simulink model "MontajeFinal"  (R2023a)
settings: Solver=ode4  StartTime=0.0  StopTime=1527  FixedStep=Ts  RelTol=1e-3  EnableMultiTasking=on
PostLoadFcn:
  | Ts=1/200000;L=1.8e-3;w=2*pi*60;C=20e-6;
  | 
  | load('NewCycleFTP75.mat')
  | 
  | Vel=Cycle(:,1);
  | Acc=Cycle(:,2);
InitFcn:
  | Ts=1/200000;L=1.8e-3;w=2*pi*60;C=20e-6;
  | 
  | load('NewCycleFTP75.mat')
  | 
  | Vel=Cycle(:,1);
  | Acc=Cycle(:,2);
values from neighbouring files (symbols this model uses):
  Cycle = [0 0 0 0 0 0 0 0 0 0 0 0 ... (4948 elements, 2474x2)]    [CycleFTP75.mat]    (also in CycleOntibon.mat = [0 0 0 0 0 0 0 0 0 0 0 0 ... (3602 elements, 1801x2)])
undefined symbols (not defined in the file or in its folder): DiscIntNeverNeededParam, sizecont
libraries: simulink x10, spsSeriesRLCBranchLib x8, spsIGBTDiodeLib x6, spsCurrentMeasurementLib x4, spsVoltageMeasurementLib x4, spsGroundLib x4, dspswit3 x2, spsDCVoltageSourceLib x1, spsAsynchronousMachineSIUnitsLib x1, spspowerguiLib x1, slpidlib x1
(part 1 of 2)
Description:
  | Model of a simple control system for use iin training.
settings Model: SimulationMode=accelerator  Creator=Paul Baracos  LastModifiedBy=Julian
settings SolverCC: AlgebraicLoopSolver=TrustRegion
settings DataIOCC: LimitDataPoints=on  SaveFormat=Array  SignalLoggingSaveFormat=ModelDataLogs  SaveOutput=off  SaveTime=off  ReturnWorkspaceOutputs=off  SignalLoggingName=sigsOut
settings OptimizationCC: BlockReduction=off  BooleanDataType=off  OptimizeBlockIOStorage=off  BufferReuse=off  ReuseModelBlockBuffer=off  GlobalBufferReuse=off  ExpressionFolding=off  LocalBlockOutputs=off  InitFltsAndDblsToZero=on  LifeSpan=inf
settings DebuggingCC: SaveWithParameterizedLinksMsg=none  UnderspecifiedInitializationDetection=Classic  MergeDetectMultiDrivingBlocksExec=none  SignalResolutionControl=TryResolveAllWithWarning  MultiTaskDSMMsg=warning  MultiTaskCondExecSysMsg=none  FcnCallInpInsideContextMsg=warning  UnconnectedInputMsg=warning  UnconnectedOutputMsg=warning  UnconnectedLineMsg=warning  SFUnexpectedBacktrackingDiag=warning  SFNoUnconditionalDefaultTransitionDiag=warning  SFExecutionAtInitializationDiag=none  ArithmeticOperatorsInVariantConditions=warning
settings HardwareCC: ProdBitPerPointer=32  ProdBitPerSizeT=32  ProdBitPerPtrDiffT=32  ProdLargestAtomicFloat=None  ProdIntDivRoundTo=Undefined  ProdEndianess=Unspecified  ProdWordSize=32  ProdHWDeviceType=32-bit Generic  TargetUnknown=on
settings ModelReferenceCC: EnableRefExpFcnMdlSchedulingChecks=on  PropagateSignalLabelsOutOfModel=off
settings SFSimCC: SimUseLocalCustomCode=off  CustomCodeUndefinedFunction=UseInterfaceOnly
settings RTWCC: RTWUseLocalCustomCode=off
settings CodeAppCC: StateflowObjectComments=on
settings GRTTargetCC: TargetFcnLib=ansi_tfl_tmw.mat  TargetLangStandard=C89/C90 (ANSI)  CombineOutputUpdateFcns=off  GRTInterface=on
settings ConfigComp: CovMetricSettings=dw  CovSaveCumulativeToWorkspaceVar=on  CovSaveSingleToWorkspaceVar=on  CovExternalEMLEnable=off
settings SimscapeCC: SimscapeNormalizeSystem=off

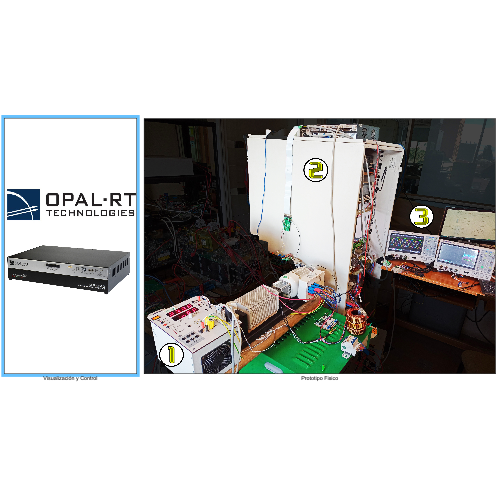
[thumbnail: Simulink's stored preview of the top-level diagram]
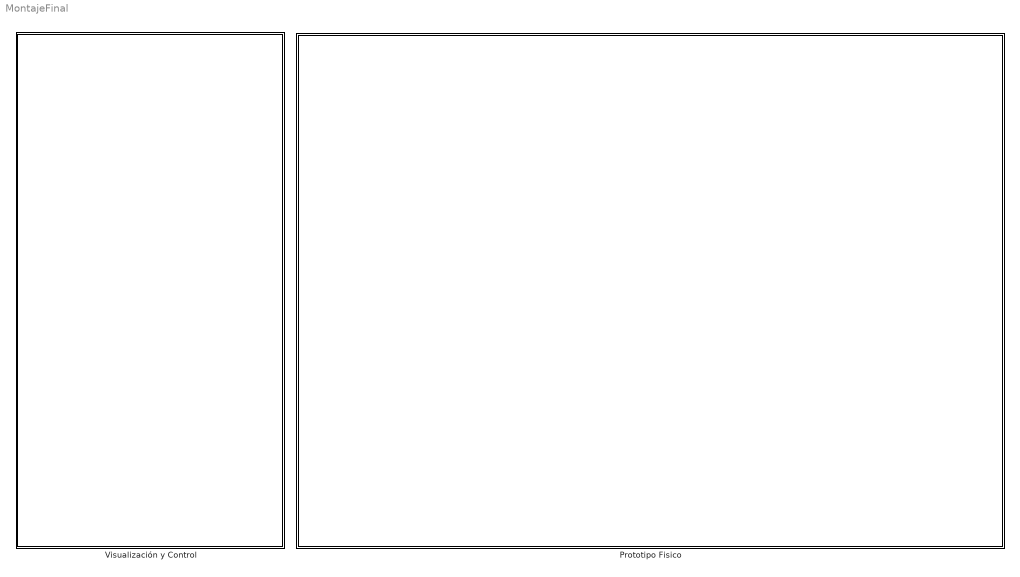
== system MontajeFinal ==
  Prototipo Fisico : Subsystem
      mask Display: image('General.jpg'); % Use "Edit Image" on toolstrip to change.
  Visualización y Control : Subsystem
      mask Display: image('Opal.jpg'); % Use "Edit Image" on toolstrip to change.

== system MontajeFinal/Prototipo Fisico ==
  Fuente Bidireccional : Subsystem
      mask Display: image('Fuente.jpg'); % Use "Edit Image" on toolstrip to change.
  Inversor - Filtro LC - Sensores : Subsystem
      mask Display: image('Sensores.jpg'); % Use "Edit Image" on toolstrip to change.
  Maquina Pendular & MIJA : Subsystem
      mask Display: image('Maquinas.jpg'); % Use "Edit Image" on toolstrip to change.
  Modulo Comunicación : Subsystem
      settings: PortSchema="{\"entries\":[{\"content\":{\"sides\":[{\"content\":{\"connectorIds\":[\"Out2\",\"In1\"]},\"type\":\"ConnectorPlacement.EquallySpacedRectSide\",\"uuid\":\"66e5c735-c63b-4ba9-ad41-caef14ec7bf0\"},{\"content\":{\"connectorIds\":[\"In2\",\"Out1\"],\"side\":\"RIGHT\"},\"type\":\"ConnectorPlacement.EquallySpacedRectSide\",\"uuid\":\"f3b04e68-f383-44b7-b279-598a5bf2e637\"},{\"content\":{\"side\":\"TOP\"},\"type\":\"ConnectorPlacement.EquallySpacedRectSide\",\"uuid\":\"c3216178-39f9-4474-948a-42e4050edd7e\"}]},\"type\":\"ConnectorPlacement.EquallySpacedConnector\",\"uuid\":\"a4194594-47fb-4665-9fd1-3f005c2be821\"}],\"packageUris\":[\"http://schema.mathworks.com/mf0/Connector/R2020b\"],\"version\":\"1.0\"}"
      mask Display: image('G:\Mi unidad\VEHICULO ELECTRICO\Articulos\Simposios\Sicel\Imagenes\Final\Comunicacion.jpg'); % Use "Edit Image" on toolstrip to change.
  powergui : spspowerguiLib/powergui  Priority=1  SimulationMode=Discrete  SampleTime=Ts  frequency=60  Iterations=50  frequencyindice=0  Pbase=100e6  ErrMax=1e-4  UnitsV=kV  UnitsW=MW  buscounter=0  FunctionMessages=off  echomessages=off  EnableUseOfTLC=off  CurrentSourceSwitches=off  DisableSnubberDevices=off  DisableRonSwitches=off  DisableVfSwitches=off  DisplayEquations=off  AutomaticDiscreteSolvers=off  SolverType=Tustin/Backward Euler (TBE)  Interpol=off  ExternalGateDelay=off  methode=off  Ts=100  x0status=blocks  SPID=on  SwTol=0  HookPort=off  NonlinearTolerance=1e-4  nMaxIteration=100  ContinueOnMaxIteration=off  RestoreLinks=warning  ResistiveCurrentMeasurement=off  Frange=[0:2:500]  Ylog=off  Xlog=on  ShowGrid=off  save=off  variable=ZData  structure=0  ZoomFFT=off  StartTime=0.0  cycles=1  DisplayStyle=1  fundamental=60  FreqAxis=off  MaxFrequency=1000  frequencyindicesteady=1  RmsSteady=1  display=off
  tag scope: Velocidad=global
  wires:
  Modulo Comunicación/1(Par_Out) -> Maquina Pendular & MIJA/1(Par)
  Modulo Comunicación/2(Vel_Out) -> [Velocidad]
  [Par] -> Modulo Comunicación/1(Par_In)
  Maquina Pendular & MIJA/1(Velocidad) -> Modulo Comunicación/2(Vel_In)
  connections:
  Fuente Bidireccional/RConn1 -- Inversor - Filtro LC - Sensores/LConn1
  Inversor - Filtro LC - Sensores/RConn2 -- Maquina Pendular & MIJA/LConn2
  Inversor - Filtro LC - Sensores/RConn3 -- Maquina Pendular & MIJA/LConn3
  Fuente Bidireccional/RConn2 -- Inversor - Filtro LC - Sensores/LConn2
  Inversor - Filtro LC - Sensores/RConn1 -- Maquina Pendular & MIJA/LConn1

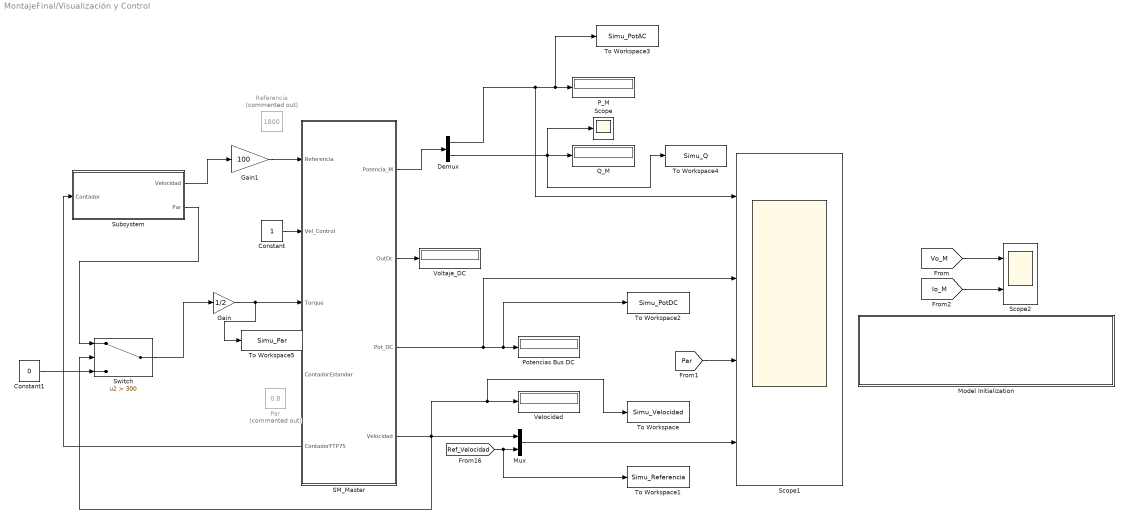
== system MontajeFinal/Visualización y Control ==
  Constant : Constant
  Constant1 : Constant  Value=0
  Demux : Demux  Outputs=2
  Gain : Gain  Gain=1/2
  Gain1 : Gain  Gain=100  SaturateOnIntegerOverflow=on  OutDataTypeStr=Inherit: Same as input  ParamDataTypeStr=Inherit: Same as input
  Model Initialization : Subsystem  AncestorBlock=artemis/Tools /Misc/Model Initialization  mask(Model Functions){InitFcnX=|, prel=off, posl=on, inif=on, strf=off}
      mask InitFcnX=|
      | Ts=1/200000;L=1.8e-3;w=2*pi*60;C=20e-6;
      |
      | load('NewCycleFTP75.mat')
      |
      | Vel=Cycle(:,1);
      | Acc=Cycle(:,2);
      mask prompts: InitFcnX "Initialisation"; prel "Preload Function"; posl "PostLoad Function"; inif "InitFcn"; strf "StartFcn"
      mask init:
      | currentBlock = gcb;
      | root = bdroot(currentBlock);
      | 
      | if ~strcmp(get_param(root,'BlockDiagramType'),'library')
      |     if prel==1
      |         set_param(root, 'PreLoadFcn', InitFcnX);
      |     else
      |         set_param(root, 'PreLoadFcn', '');
      |     end
      |     if inif==1
      |         set_param(root, 'InitFcn', InitFcnX);
      |     else
      |         set_param(root, 'InitFcn', '');
      |     end
      |     if strf==1
      |         set_param(root, 'StartFcn', InitFcnX);
      |     else
      |         set_param(root, 'StartFcn', '');
      |     end
      |     if posl==1
      |         set_param(root, 'PostLoadFcn', InitFcnX);
      |     else
      |         set_param(root, 'PostLoadFcn', '');
      |     end
      | end
      | 
      | pos = get_param(currentBlock, 'Position');
      | width = pos(3) - pos(1); height = pos(4) - pos(2);
      | txt = [ upper(root) '\n' '- InitFcn. . . . . '  get_param(root, 'InitFcn') ];
      settings: LibrarySourceBlock=artemis/Tools /Misc/Model Initialization  CopyFcn=set_param(gcb,'LinkStatus','inactive')
      mask Display: text(5, height*0.5, txt, 'horizontalAlignment', 'left', 'verticalAlignment', 'middle') ;
  Mux : Mux  Inputs=2
  P_M : Display
  Par : Constant  Commented=on  Value=0.8
  Potencias Bus DC : Display
  Q_M : Display
  Referencia : Constant  Commented=on  Value=1800
  SM_Master : Subsystem
      settings: PortSchema="{\"entries\":[{\"content\":{\"sides\":[{\"content\":{\"connectorIds\":[\"In1\",\"In2\",\"In3\",\"Out5\",\"Out6\"]},\"type\":\"ConnectorPlacement.EquallySpacedRectSide\",\"uuid\":\"2bfde8e4-db29-467b-a3e6-219bd979e2b6\"},{\"content\":{\"connectorIds\":[\"Out1\",\"Out2\",\"Out3\",\"Out4\"],\"side\":\"RIGHT\"},\"type\":\"ConnectorPlacement.EquallySpacedRectSide\",\"uuid\":\"a7f0eab7-0a0b-47e1-a185-527893d455d2\"},{\"content\":{\"side\":\"TOP\"},\"type\":\"ConnectorPlacement.EquallySpacedRectSide\",\"uuid\":\"1aba6232-4c2d-4fe6-89ed-3e8cc09b7475\"}]},\"type\":\"ConnectorPlacement.EquallySpacedConnector\",\"uuid\":\"12a0442f-195f-492e-b9e3-ea8deb1e0ede\"}],\"packageUris\":[\"http://schema.mathworks.com/mf0/Connector/R2020b\"],\"version\":\"1.0\"}"
  Scope : Scope
  Scope1 : Scope  NumInputPorts=4
  Scope2 : Scope  NumInputPorts=2
  Subsystem : Subsystem
  Switch : Switch  Criteria=u2 > Threshold  Threshold=300  SaturateOnIntegerOverflow=off  InputSameDT=off
  To Workspace : ToWorkspace  VariableName=Simu_Velocidad  SampleTime=1/2000
      settings: Save2DSignal=2-D array (concatenate along first dimension)
  To Workspace1 : ToWorkspace  VariableName=Simu_Referencia  SampleTime=1/2000
      settings: Save2DSignal=2-D array (concatenate along first dimension)
  To Workspace2 : ToWorkspace  VariableName=Simu_PotDC  SampleTime=1/2000
      settings: Save2DSignal=2-D array (concatenate along first dimension)
  To Workspace3 : ToWorkspace  VariableName=Simu_PotAC  SampleTime=1/2000
      settings: Save2DSignal=2-D array (concatenate along first dimension)
  To Workspace4 : ToWorkspace  VariableName=Simu_Q  SampleTime=1/2000
      settings: Save2DSignal=2-D array (concatenate along first dimension)
  To Workspace5 : ToWorkspace  VariableName=Simu_Par  SampleTime=1/2000
      settings: Save2DSignal=2-D array (concatenate along first dimension)
  Velocidad : Display
  Voltaje_DC : Display
  wires:
  SM_Master/1(Potencia_M) -> Demux/1
  Demux/2 -> To Workspace4/1, Scope/1, Q_M/1
  Demux/1 -> Scope1/1, To Workspace3/1, P_M/1
  SM_Master/2(OutDc) -> Voltaje_DC/1
  Constant/1 -> SM_Master/2(Vel_Control)
  SM_Master/3(Pot_DC) -> To Workspace2/1, Potencias Bus DC/1, Scope1/2
  SM_Master/4(Velocidad) -> Switch/2, To Workspace/1, Velocidad/1, Mux/1
  [Ref_Velocidad] -> To Workspace1/1, Mux/2
  [Vo_M] -> Scope2/1
  [Io_M] -> Scope2/2
  [Par] -> Scope1/3
  Mux/1 -> Scope1/4
  Gain/1 -> To Workspace5/1, SM_Master/3(Torque)
  SM_Master/6(ContadorFTP75) -> Subsystem/1(Contador)
  Gain1/1 -> SM_Master/1(Referencia)
  Subsystem/1(Velocidad) -> Gain1/1
  Switch/1 -> Gain/1
  Constant1/1 -> Switch/3
  Subsystem/2(Par) -> Switch/1

== system MontajeFinal/Prototipo Fisico/Fuente Bidireccional ==
  Current Measurement3 : spsCurrentMeasurementLib/Current Measurement  PhasorSimulation=off  OutputType=Complex  PSBequivalent=0
  DC Voltage Source : spsDCVoltageSourceLib/DC Voltage Source  Amplitude=1000  Measurements=None
  Series RLC Branch6 : spsSeriesRLCBranchLib/Series RLC Branch  LConnTagsString=__new0  RConnTagsString=__new0  BranchType=C  Resistance=0.0000000000000000000000000000000000000000000001  Inductance=L  SetiL0=off  InitialCurrent=0  Capacitance=0.1  Setx0=off  InitialVoltage=0  Measurements=None
  Series RLC Branch7 : spsSeriesRLCBranchLib/Series RLC Branch  LConnTagsString=__new0  RConnTagsString=__new0  BranchType=R  Resistance=0.1  Inductance=L  SetiL0=off  InitialCurrent=0  Capacitance=0.001  Setx0=off  InitialVoltage=0  Measurements=None
  Voltage Measurement4 : spsVoltageMeasurementLib/Voltage Measurement  PhasorSimulation=off  OutputType=Complex  PSBequivalent=0
  + : PMIOPort  Side=Right
  - : PMIOPort  Port=2  Side=Right
  tag scope: Idc=global, Vdc=global
  wires:
  Voltage Measurement4/1 -> [Vdc]
  Current Measurement3/1 -> [Idc]
  connections:
  Series RLC Branch7/LConn1 -- Series RLC Branch6/LConn1 -- Voltage Measurement4/LConn1 -- +/RConn1
  Series RLC Branch6/RConn1 -- DC Voltage Source/LConn1 -- -/RConn1 -- Voltage Measurement4/LConn2
  Series RLC Branch7/RConn1 -- Current Measurement3/RConn1
  Current Measurement3/LConn1 -- DC Voltage Source/RConn1

== system MontajeFinal/Prototipo Fisico/Inversor - Filtro LC - Sensores ==
  Filtro LC & Sensores : Subsystem
  Inversor : Subsystem
  a : PMIOPort  Side=Right
  Vdc : PMIOPort  Port=2  Side=Left
  b : PMIOPort  Port=3  Side=Right
  -Vdc : PMIOPort  Port=4  Side=Left
  c : PMIOPort  Port=5  Side=Right
  connections:
  Filtro LC & Sensores/LConn3 -- Inversor/RConn3
  Filtro LC & Sensores/LConn1 -- Inversor/RConn1
  Filtro LC & Sensores/RConn2 -- b/RConn1
  Filtro LC & Sensores/LConn2 -- Inversor/RConn2
  Filtro LC & Sensores/RConn1 -- a/RConn1
  Filtro LC & Sensores/RConn3 -- c/RConn1
  -Vdc/RConn1 -- Inversor/LConn2
  Vdc/RConn1 -- Inversor/LConn1

== system MontajeFinal/Prototipo Fisico/Maquina Pendular & MIJA ==
  Par : Inport
  Bus Selector : BusSelector  OutputSignals=Mechanical.Rotor speed (wm)
  Gain : Gain  Gain=30/pi
  MIJA : spsAsynchronousMachineSIUnitsLib/Asynchronous Machine SI Units  RotorType=Squirrel-cage  PresetModel=No  MechanicalLoad=Torque Tm  ShowDetailedParameters=on  ReferenceFrame=Rotor  Units=SI  MeasurementBus=off  NominalParameters=[250 230 50]  VoltageRatio=1  Stator=[45.50 0.20]  Rotor=[20 0.04]  Cage1=[0.4155 0.002066]  Cage2=[0.4168 0.0003495]  Lm=1.08  Mechanical=[0.003 0.00112 2]  PolePairs=2  InitialConditions=[1 0 0 0 0 0 0 0]  SimulateSaturation=off  Saturation=[14.03593122, 27.81365428, 53.79336849, 72.68890987, 97.98006896, 148.6815601, 215.7428561, 302.9841135, 428.7778367 ; 230, 322, 414, 460, 506, 552, 598, 644, 690]  LoadFlowParameters=1492000  TsPowergui=0  TsBlock=-1  IterativeModel=Trapezoidal non iterative  IterativeDiscreteModel=Trapezoidal non iterative  Pmec=250
  A : PMIOPort  Side=Left
  B : PMIOPort  Port=2  Side=Left
  C : PMIOPort  Port=3  Side=Left
  Velocidad : Outport
  wires:
  Gain/1 -> Velocidad/1
  Bus Selector/1 -> Gain/1  "<Rotor speed (wm)>"
  MIJA/1 -> Bus Selector/1
  Par/1 -> MIJA/1
  connections:
  B/RConn1 -- MIJA/LConn2
  C/RConn1 -- MIJA/LConn3
  A/RConn1 -- MIJA/LConn1

== system MontajeFinal/Prototipo Fisico/Modulo Comunicación ==
  Par_In : Inport
  Vel_In : Inport  Port=2
  Gain : Gain
  Gain2 : Gain
  Par_Out : Outport
  Vel_Out : Outport  Port=2
  wires:
  Gain/1 -> Vel_Out/1
  Gain2/1 -> Par_Out/1
  Par_In/1 -> Gain2/1
  Vel_In/1 -> Gain/1

== system MontajeFinal/Visualización y Control/Model Initialization ==

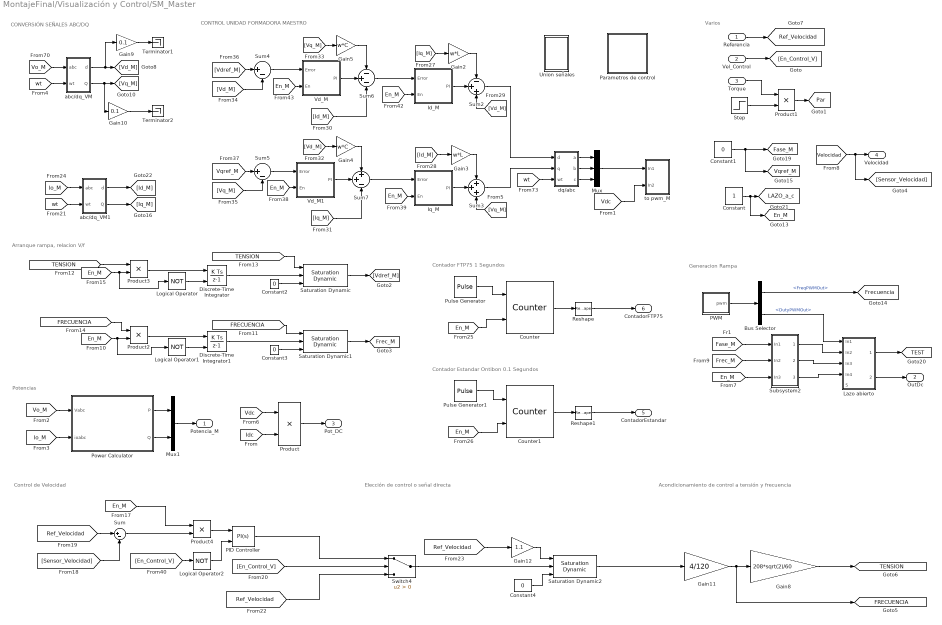
== system MontajeFinal/Visualización y Control/SM_Master ==
  note: Varios
  note: Generacion Rampa
  note: Potencias
  note: CONVERSIÓN SEÑALES ABC/DQ
  note: CONTROL UNIDAD FORMADORA MAESTRO
  note: Arranque rampa, relacion V/f
  note: Elección de control o señal directa
  note: Acondicionamiento de control a tensión y frecuencia
  note: Control de Velocidad
  note: Contador FTP75 1 Segundos
  note: Contador Estandar Ontibon 0.1 Segundos
  Referencia : Inport
  Vel_Control : Inport  Port=2
  Torque : Inport  Port=3
  Bus Selector : BusSelector  OutputSignals=FreqPWMOut,DutyPWMOut
  Constant : Constant
  Constant{1..4} (4 alike) : Constant  Value=0
  Counter : dspswit3/Counter  Direction=Up  CountEvent=Rising edge  CounterSize=User defined  MaxCount=2474  InitialCount=0  Output=Count  HitValue=sizecont-1  ResetInput=on  SamplesPerFrame=1  Ts=1  CntDtype=double  HitDtype=Logical
  Counter1 : dspswit3/Counter  Direction=Up  CountEvent=Rising edge  CounterSize=User defined  MaxCount=2474  InitialCount=0  Output=Count  HitValue=sizecont-1  ResetInput=on  SamplesPerFrame=1  Ts=1  CntDtype=double  HitDtype=Logical
  Discrete-Time Integrator : DiscreteIntegrator  ExternalReset=level  SampleTime=-1  ICPrevOutput=DiscIntNeverNeededParam  ICPrevScaledInput=DiscIntNeverNeededParam
  Discrete-Time Integrator1 : DiscreteIntegrator  ExternalReset=level  SampleTime=-1  ICPrevOutput=DiscIntNeverNeededParam  ICPrevScaledInput=DiscIntNeverNeededParam
  Gain10 : Gain  Gain=0.1
  Gain11 : Gain  Gain=4/120
  Gain12 : Gain  Gain=1.1
  Gain2 : Gain  Gain=w*L
  Gain3 : Gain  Gain=w*L
  Gain4 : Gain  Gain=w*C
  Gain5 : Gain  Gain=w*C
  Gain8 : Gain  Gain=208*sqrt(2)/60  SaturateOnIntegerOverflow=on  OutDataTypeStr=Inherit: Same as input  ParamDataTypeStr=Inherit: Same as input
  Gain9 : Gain  Gain=0.1
  Id_M : Subsystem
  Iq_M : Subsystem
  "Lazo abierto " : Subsystem
  Logical Operator : Logic  Operator=NOT  AllPortsSameDT=off  OutDataTypeStr=boolean
  Logical Operator1 : Logic  Operator=NOT  AllPortsSameDT=off  OutDataTypeStr=boolean
  Logical Operator2 : Logic  Operator=NOT  AllPortsSameDT=off  OutDataTypeStr=boolean
  Mux : Mux  Inputs=3
  Mux1 : Mux  Inputs=2
  PID Controller : slpidlib/PID Controller  Controller=PI  Form=Parallel  TimeDomain=Continuous-time  UseExternalTs=off  SampleTime=-1  IntegratorMethod=Forward Euler  FilterMethod=Forward Euler  ControllerParametersSource=internal  P=0.502  I=21.7  UseKiTs=off  D=0  N=100  UseFilter=on  TunerSelectOption=Transfer Function Based (PID Tuner App)  InitialConditionSource=internal  InitialConditionForIntegrator=0  InitialConditionForFilter=0  DifferentiatorICPrevScaledInput=0  ExternalReset=level  TrackingMode=off  Kt=1  LimitOutput=off  SatLimitsSource=internal  UpperSaturationLimit=inf  LowerSaturationLimit=-inf  LinearizeAsGain=on  AntiWindupMode=none  Kb=1  LimitIntegrator=off  UpperIntegratorSaturationLimit=inf  LowerIntegratorSaturationLimit=-inf  POutMin=[]  POutMax=[]  IOutMin=[]  IOutMax=[]  DOutMin=[]  DOutMax=[]  NOutMin=[]  NOutMax=[]  SumOutMin=[]  SumOutMax=[]  SaturationOutMin=[]  SaturationOutMax=[]  PParamMin=[]  PParamMax=[]  IParamMin=[]  IParamMax=[]  DParamMin=[]  DParamMax=[]  NParamMin=[]  NParamMax=[]  KbParamMin=[]  KbParamMax=[]  KtParamMin=[]  KtParamMax=[]  KbOutMin=[]  KbOutMax=[]  KtOutMin=[]  KtOutMax=[]  IntegratorOutMin=[]  IntegratorOutMax=[]  FilterOutMin=[]  FilterOutMax=[]  SumI1OutMin=[]  SumI1OutMax=[]  SumI2OutMin=[]  SumI2OutMax=[]  SumI3OutMin=[]  SumI3OutMax=[]  SumI4OutMin=[]  SumI4OutMax=[]  SumDOutMin=[]  SumDOutMax=[]  DifferentiatorOutMin=[]  DifferentiatorOutMax=[]  FilterDiffOutCoefMin=[]  FilterDiffOutCoefMax=[]  ReciprocalOutMin=[]  ReciprocalOutMax=[]  SumDenOutMin=[]  SumDenOutMax=[]  SumNumOutMin=[]  SumNumOutMax=[]  DivideOutMin=[]  DivideOutMax=[]  UdiffTsProdOutMin=[]  UdiffTsProdOutMax=[]  NTsProdOutMin=[]  NTsProdOutMax=[]  UintegralTsProdOutMin=[]  UintegralTsProdOutMax=[]  UngainTsProdOutMin=[]  UngainTsProdOutMax=[]  ClampingZeroOutDataTypeStr=Inherit: Inherit via back propagation  ClampingZeroOutMin=[]  ClampingZeroOutMax=[]  FilterDenConstantOutDataTypeStr=Inherit: Inherit via back propagation  FilterDenConstantOutMin=[]  FilterDenConstantOutMax=[]  PCopyOutDataTypeStr=Inherit: Inherit via back propagation  PCopyOutMin=[]  PCopyOutMax=[]  NCopyOutDataTypeStr=Inherit: Inherit via back propagation  NCopyOutMin=[]  NCopyOutMax=[]  IntegratorContinuousStateAttributes=''  IntegratorStateMustResolveToSignalObject=off  IntegratorRTWStateStorageClass=Auto  FilterContinuousStateAttributes=''  FilterStateMustResolveToSignalObject=off  FilterRTWStateStorageClass=Auto  ParallelPVariant=InternalParameters  IdealPVariant=Disabled  IVariant=InternalParameters  DVariant=Disabled  IntegratorVariant=Continuous  SatVariant=Disabled  AWVariant=Passthrough  PCopyVariant=Disabled  TRVariant=Disabled  FdbkBlocksVariant=Forward  IdealPFdbkVariant=Disabled  SatFdbkVariant=Disabled  DerivativeFilterVariant=Disabled  NVariant=Disabled  NCopyVariant=Disabled_SignalSpec  FilterICVariant=Disabled  IntegratorICVariant=InternalICs  ExternalResetVariant=ExternalReset  TRSumVariant=Passthrough  SumFdbkVariant=Disabled  SumVariant=Sum_PI  TsampFilterVariant=InternalTs  TsampNgainVariant=Passthrough  TsampIntegralVariant=Disabled_SignalSpec  ExternalSaturationOutDataTypeStr=Inherit: Same as second input
  PWM : Subsystem
  Parametros de control : Subsystem
  Power Calculator : Subsystem
  Product{,1..4} (5 alike) : Product
  Pulse Generator : DiscretePulseGenerator  PulseType=Time based  Period=1  PulseWidth=5
  Pulse Generator1 : DiscretePulseGenerator  PulseType=Time based  Period=0.1  PulseWidth=5
  Reshape : Reshape  OutputDimensionality=Customize  OutputDimensions=[1]
  Reshape1 : Reshape  OutputDimensionality=Customize  OutputDimensions=[1]
  Saturation Dynamic : simulink/Discontinuities/Saturation Dynamic  OutMin=[]  OutMax=[]  OutDataTypeStr=Inherit: Same as second input  OutDataType=fixdt(1, 16)  OutScaling=2^-10  DoSatur=off
  Saturation Dynamic1 : simulink/Discontinuities/Saturation Dynamic  OutMin=[]  OutMax=[]  OutDataTypeStr=Inherit: Same as second input  OutDataType=fixdt(1, 16)  OutScaling=2^-10  DoSatur=off
  Saturation Dynamic2 : simulink/Discontinuities/Saturation Dynamic  OutMin=[]  OutMax=[]  OutDataTypeStr=Inherit: Same as second input  OutDataType=fixdt(1, 16)  OutScaling=2^-10  DoSatur=off
  Step : Step  Time=0.2  SampleTime=0
  Subsystem2 : Subsystem
  Sum : Sum  Inputs=|+-
  Sum2 : Sum  Inputs=-++
  Sum3 : Sum  Inputs=+++
  Sum4 : Sum  Inputs=|+-
  Sum5 : Sum  Inputs=|+-
  Sum6 : Sum  Inputs=-+-
  Sum7 : Sum  Inputs=++-
  Switch4 : Switch  Criteria=u2 > Threshold  SaturateOnIntegerOverflow=off  InputSameDT=off
  Terminator1 : Terminator
  Terminator2 : Terminator
  "Union señales " : Subsystem
  Vd_M : Subsystem
  Vd_M1 : Subsystem
  abc/dq_VM : Subsystem
  abc/dq_VM1 : Subsystem
  dq/abc : Subsystem
  to pwm_M : Subsystem
  Potencia_M : Outport
  OutDc : Outport  Port=2
  Pot_DC : Outport  Port=3
  Velocidad : Outport  Port=4
  ContadorEstandar : Outport  Port=5
  ContadorFTP75 : Outport  Port=6
  tag scope: En_M=global, FRECUENCIA=global, Fase_M=global, Frec_M=global, Frecuencia=global, LAZO_a_c=global, Par=global, Ref_Velocidad=global, TENSION=global, TEST=global, Vqref_M=global
  wires:
  [Vo_M] -> abc/dq_VM/1(abc)
  abc/dq_VM1/1(d) -> [Id_M]
  [Io_M] -> abc/dq_VM1/1(abc)
  abc/dq_VM/2(Q) -> Gain10/1, [Vq_M]
  [wt] -> abc/dq_VM1/2(wt)
  [wt] -> abc/dq_VM/2(wt)
  abc/dq_VM1/2(Q) -> [Iq_M]
  abc/dq_VM/1(d) -> Gain9/1, [Vd_M]
  Gain5/1 -> Sum6/1
  Gain3/1 -> Sum3/1
  [Id_M] -> Gain3/1
  [Vdref_M] -> Sum4/1
  [Vq_M] -> Sum3/3
  Sum7/1 -> Iq_M/1(Error)
  [Id_M] -> Sum6/3
  [Vd_M] -> Gain4/1
  [En_M] -> Vd_M1/2(En)
  [Vq_M] -> Sum5/2
  Sum2/1 -> dq/abc/1(d)
  [En_M] -> Vd_M/2(En)
  dq/abc/3(c) -> Mux/3
  [Iq_M] -> Sum7/3
  [En_M] -> Iq_M/2(En)
  Gain2/1 -> Sum2/1
  [Vq_M] -> Gain5/1
  dq/abc/2(b) -> Mux/2
  dq/abc/1(a) -> Mux/1
  [wt] -> dq/abc/3(wt)
  Gain4/1 -> Sum7/1
  Sum3/1 -> dq/abc/2(q)
  [Vd_M] -> Sum4/2
  Sum5/1 -> Vd_M1/1(Error)
  Id_M/1(PI) -> Sum2/2
  Sum6/1 -> Id_M/1(Error)
  [Vd_M] -> Sum2/3
  Sum4/1 -> Vd_M/1(Error)
  [Iq_M] -> Gain2/1
  Vd_M/1(PI) -> Sum6/2
  Iq_M/1(PI) -> Sum3/2
  [En_M] -> Id_M/2(En)
  [Vqref_M] -> Sum5/1
  Vd_M1/1(PI) -> Sum7/2
  [Vdc] -> to pwm_M/2(In2)
  Gain9/1 -> Terminator1/1
  [Vo_M] -> Power Calculator/1(Vabc)
  [Io_M] -> Power Calculator/2(ioabc)
  Power Calculator/2("Q ") -> Mux1/2
  Power Calculator/1(P) -> Mux1/1
  Mux1/1 -> Potencia_M/1
  Gain10/1 -> Terminator2/1
  Mux/1 -> to pwm_M/1(In1)
  Bus Selector/1 -> [Frecuencia]  "<FreqPWMOut>"
  [Fase_M] -> Subsystem2/1(In1)
  Subsystem2/1(Out1) -> "Lazo abierto "/2(In2)
  "Lazo abierto "/2(Out2) -> OutDc/1
  "Lazo abierto "/1(Out1) -> [TEST]
  Subsystem2/2(Out2) -> "Lazo abierto "/3(In3)
  Subsystem2/3(Out3) -> "Lazo abierto "/4(In4)
  [En_M] -> Subsystem2/3(In3)
  Bus Selector/2 -> "Lazo abierto "/1(In1)  "<DutyPWMOut>"
  [Frec_M] -> Subsystem2/2(In2)
  PWM/1("pwm ") -> Bus Selector/1
  Constant/1 -> [En_M], [LAZO_a_c]
  [Idc] -> Product/2
  [Vdc] -> Product/1
  Product/1 -> Pot_DC/1
  Constant1/1 -> [Vqref_M], [Fase_M]
  [Velocidad] -> [Sensor_Velocidad], Velocidad/1
  Referencia/1 -> [Ref_Velocidad]
  Vel_Control/1 -> [En_Control_V]
  Step/1 -> Product1/2
  Torque/1 -> Product1/1
  Product1/1 -> [Par]
  Logical Operator/1 -> Discrete-Time Integrator/2
  [En_M] -> Logical Operator/1, Product3/2
  Product3/1 -> Discrete-Time Integrator/1
  [FRECUENCIA] -> Product2/1
  Saturation Dynamic/1 -> [Vdref_M]
  [En_M] -> Logical Operator1/1, Product2/2
  Constant2/1 -> Saturation Dynamic/3
  [TENSION] -> Product3/1
  Logical Operator1/1 -> Discrete-Time Integrator1/2
  [TENSION] -> Saturation Dynamic/1
  Discrete-Time Integrator/1 -> Saturation Dynamic/2
  Discrete-Time Integrator1/1 -> Saturation Dynamic1/2
  Constant3/1 -> Saturation Dynamic1/3
  [FRECUENCIA] -> Saturation Dynamic1/1
  Product2/1 -> Discrete-Time Integrator1/1
  Saturation Dynamic1/1 -> [Frec_M]
  Switch4/1 -> Saturation Dynamic2/2
  [En_Control_V] -> Switch4/2
  [Ref_Velocidad] -> Gain12/1
  PID Controller/1 -> Switch4/1
  [Ref_Velocidad] -> Sum/1
  Constant4/1 -> Saturation Dynamic2/3
  Gain11/1 -> Gain8/1, [FRECUENCIA]
  Product4/1 -> PID Controller/1
  Gain12/1 -> Saturation Dynamic2/1
  Gain8/1 -> [TENSION]
  Sum/1 -> Product4/2
  [En_M] -> Product4/1
  Logical Operator2/1 -> PID Controller/2
  Saturation Dynamic2/1 -> Gain11/1
  [Ref_Velocidad] -> Switch4/3
  [Sensor_Velocidad] -> Sum/2
  [En_M] -> Counter1/2
  Pulse Generator/1 -> Counter/1
  Reshape/1 -> ContadorFTP75/1
  Reshape1/1 -> ContadorEstandar/1
  [En_M] -> Counter/2
  Pulse Generator1/1 -> Counter1/1
  Counter1/1 -> Reshape1/1
  Counter/1 -> Reshape/1
  [En_Control_V] -> Logical Operator2/1

== system MontajeFinal/Visualización y Control/Subsystem ==
  Contador : Inport
  Constant1 : Constant  Value=Acc
  Constant3 : Constant  Value=Vel
  Index Vector1 : MultiPortSwitch  DataPortOrder=Zero-based contiguous  Inputs=1  zeroidx=on  SaturateOnIntegerOverflow=off  InputSameDT=off
  Index Vector2 : MultiPortSwitch  DataPortOrder=Zero-based contiguous  Inputs=1  zeroidx=on  SaturateOnIntegerOverflow=off  InputSameDT=off
  Reshape : Reshape  OutputDimensionality=Customize  OutputDimensions=[1]
  Reshape1 : Reshape  OutputDimensionality=Customize  OutputDimensions=[1]
  Velocidad : Outport
  Par : Outport  Port=2
  wires:
  Constant3/1 -> Index Vector2/2
  Index Vector1/1 -> Reshape1/1  "Pload1"
  Index Vector2/1 -> Reshape/1  "Pload1"
  Reshape1/1 -> Par/1
  Reshape/1 -> Velocidad/1
  Constant1/1 -> Index Vector1/2
  Contador/1 -> Index Vector2/1, Index Vector1/1

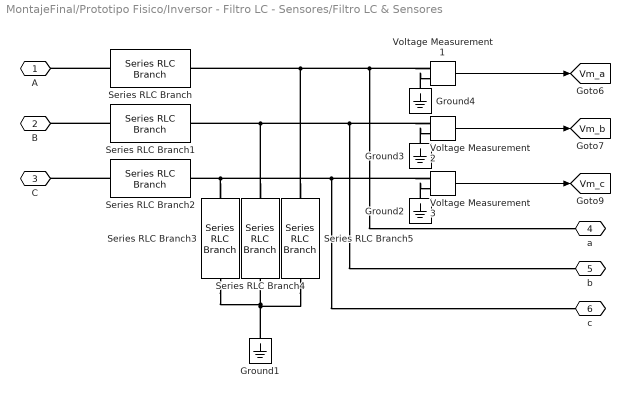
== system MontajeFinal/Prototipo Fisico/Inversor - Filtro LC - Sensores/Filtro LC & Sensores ==
  Ground{1..4} (4 alike) : spsGroundLib/Ground  LConnTagsString=a
  Series RLC Branch : spsSeriesRLCBranchLib/Series RLC Branch  LConnTagsString=__new0  RConnTagsString=__new0  BranchType=RL  Resistance=0.000001  Inductance=L  SetiL0=off  InitialCurrent=0  Capacitance=1e-6  Setx0=off  InitialVoltage=0  Measurements=None
  Series RLC Branch1 : spsSeriesRLCBranchLib/Series RLC Branch  LConnTagsString=__new0  RConnTagsString=__new0  BranchType=RL  Resistance=0.000001  Inductance=L  SetiL0=off  InitialCurrent=0  Capacitance=1e-6  Setx0=off  InitialVoltage=0  Measurements=None
  Series RLC Branch2 : spsSeriesRLCBranchLib/Series RLC Branch  LConnTagsString=__new0  RConnTagsString=__new0  BranchType=RL  Resistance=0.000001  Inductance=L  SetiL0=off  InitialCurrent=0  Capacitance=1e-6  Setx0=off  InitialVoltage=0  Measurements=None
  Series RLC Branch3 : spsSeriesRLCBranchLib/Series RLC Branch  LConnTagsString=__new0  RConnTagsString=__new0  BranchType=C  Resistance=0.1  Inductance=L  SetiL0=off  InitialCurrent=0  Capacitance=C  Setx0=off  InitialVoltage=0  Measurements=None
  Series RLC Branch4 : spsSeriesRLCBranchLib/Series RLC Branch  LConnTagsString=__new0  RConnTagsString=__new0  BranchType=C  Resistance=0.1  Inductance=L  SetiL0=off  InitialCurrent=0  Capacitance=C  Setx0=off  InitialVoltage=0  Measurements=None
  Series RLC Branch5 : spsSeriesRLCBranchLib/Series RLC Branch  LConnTagsString=__new0  RConnTagsString=__new0  BranchType=C  Resistance=0.1  Inductance=L  SetiL0=off  InitialCurrent=0  Capacitance=C  Setx0=off  InitialVoltage=0  Measurements=None
  Voltage Measurement1 : spsVoltageMeasurementLib/Voltage Measurement  PhasorSimulation=off  OutputType=Complex  PSBequivalent=0
  Voltage Measurement2 : spsVoltageMeasurementLib/Voltage Measurement  PhasorSimulation=off  OutputType=Complex  PSBequivalent=0
  Voltage Measurement3 : spsVoltageMeasurementLib/Voltage Measurement  PhasorSimulation=off  OutputType=Complex  PSBequivalent=0
  A : PMIOPort  Side=Left
  B : PMIOPort  Port=2  Side=Left
  C : PMIOPort  Port=3  Side=Left
  a : PMIOPort  Port=4  Side=Right
  b : PMIOPort  Port=5  Side=Right
  c : PMIOPort  Port=6  Side=Right
  tag scope: Vm_a=global, Vm_b=global, Vm_c=global
  wires:
  Voltage Measurement3/1 -> [Vm_c]
  Voltage Measurement2/1 -> [Vm_b]
  Voltage Measurement1/1 -> [Vm_a]
  connections:
  Voltage Measurement2/LConn1 -- b/RConn1 -- Series RLC Branch4/LConn1 -- Series RLC Branch1/RConn1
  Voltage Measurement3/LConn1 -- c/RConn1 -- Series RLC Branch3/LConn1 -- Series RLC Branch2/RConn1
  Series RLC Branch1/LConn1 -- B/RConn1
  Series RLC Branch/RConn1 -- a/RConn1 -- Voltage Measurement1/LConn1 -- Series RLC Branch5/LConn1
  Series RLC Branch4/RConn1 -- Ground1/LConn1 -- Series RLC Branch5/RConn1 -- Series RLC Branch3/RConn1
  Ground2/LConn1 -- Voltage Measurement3/LConn2
  Ground3/LConn1 -- Voltage Measurement2/LConn2
  Ground4/LConn1 -- Voltage Measurement1/LConn2
  Series RLC Branch/LConn1 -- A/RConn1
  Series RLC Branch2/LConn1 -- C/RConn1

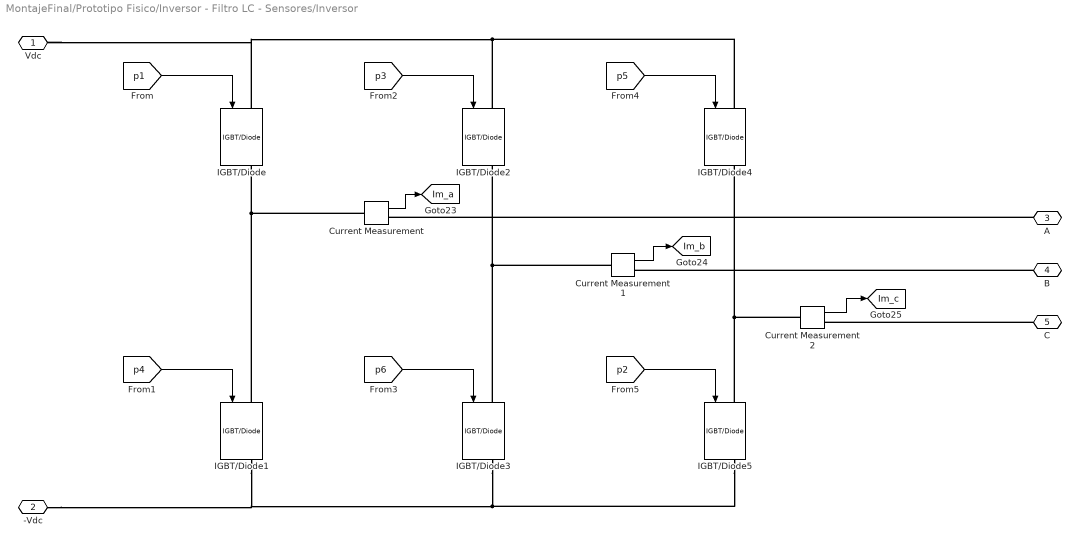
== system MontajeFinal/Prototipo Fisico/Inversor - Filtro LC - Sensores/Inversor ==
  Current Measurement : spsCurrentMeasurementLib/Current Measurement  PhasorSimulation=off  OutputType=Complex  PSBequivalent=0
  Current Measurement1 : spsCurrentMeasurementLib/Current Measurement  PhasorSimulation=off  OutputType=Complex  PSBequivalent=0
  Current Measurement2 : spsCurrentMeasurementLib/Current Measurement  PhasorSimulation=off  OutputType=Complex  PSBequivalent=0
  IGBT/Diode{,1..5} (6 alike) : spsIGBTDiodeLib/IGBT//Diode  Ron=1e-3  Rs=1e5  Cs=inf  Measurements=on
  Vdc : PMIOPort  Side=Left
  -Vdc : PMIOPort  Port=2  Side=Left
  A : PMIOPort  Port=3  Side=Right
  B : PMIOPort  Port=4  Side=Right
  C : PMIOPort  Port=5  Side=Right
  tag scope: Im_a=global, Im_b=global, Im_c=global
  wires:
  Current Measurement2/1 -> [Im_c]
  [p4] -> IGBT/Diode1/1
  [p3] -> IGBT/Diode2/1
  Current Measurement1/1 -> [Im_b]
  [p6] -> IGBT/Diode3/1
  [p5] -> IGBT/Diode4/1
  [p2] -> IGBT/Diode5/1
  [p1] -> IGBT/Diode/1
  Current Measurement/1 -> [Im_a]
  connections:
  IGBT/Diode3/RConn1 -- -Vdc/RConn1 -- IGBT/Diode1/RConn1 -- IGBT/Diode5/RConn1
  IGBT/Diode3/LConn1 -- Current Measurement1/LConn1 -- IGBT/Diode2/RConn1
  IGBT/Diode1/LConn1 -- Current Measurement/LConn1 -- IGBT/Diode/RConn1
  IGBT/Diode2/LConn1 -- IGBT/Diode/LConn1 -- Vdc/RConn1 -- IGBT/Diode4/LConn1
  IGBT/Diode5/LConn1 -- Current Measurement2/LConn1 -- IGBT/Diode4/RConn1
  B/RConn1 -- Current Measurement1/RConn1
  C/RConn1 -- Current Measurement2/RConn1
  A/RConn1 -- Current Measurement/RConn1

== system MontajeFinal/Visualización y Control/SM_Master/Id_M ==
  Error : Inport
  En : Inport  Port=2
  Constant2 : Constant  Value=0
  FF Int : DiscreteIntegrator  ExternalReset=level  InitialConditionSource=external  InitialCondition=4  SampleTime=Ts  ICPrevOutput=DiscIntNeverNeededParam  ICPrevScaledInput=DiscIntNeverNeededParam
  Logical Operator : Logic  Operator=NOT  AllPortsSameDT=off  OutDataTypeStr=boolean
  Subsystem : Subsystem
  Subsystem1 : Subsystem
  Sum3 : Sum  OutDataTypeStr=Inherit: Same as first input
  PI : Outport
  wires:
  Subsystem/1(X*Y) -> Sum3/1
  Error/1 -> Subsystem1/1(X), Subsystem/2(Y)
  [Ki_IM] -> Subsystem1/2(Y)
  [Kp_IM] -> Subsystem/1(X)
  Sum3/1 -> PI/1
  En/1 -> Logical Operator/1, Subsystem1/3(En), Subsystem/3(En)
  Logical Operator/1 -> FF Int/2
  Constant2/1 -> FF Int/3
  Subsystem1/1(X*Y) -> FF Int/1
  FF Int/1 -> Sum3/2

== system MontajeFinal/Visualización y Control/SM_Master/Iq_M ==
  Error : Inport
  En : Inport  Port=2
  Constant2 : Constant  Value=0
  FF Int : DiscreteIntegrator  ExternalReset=level  InitialConditionSource=external  InitialCondition=4  SampleTime=Ts  ICPrevOutput=DiscIntNeverNeededParam  ICPrevScaledInput=DiscIntNeverNeededParam
  Logical Operator : Logic  Operator=NOT  AllPortsSameDT=off  OutDataTypeStr=boolean
  Subsystem : Subsystem
  Subsystem1 : Subsystem
  Sum3 : Sum  OutDataTypeStr=Inherit: Same as first input
  PI : Outport
  wires:
  Subsystem/1(X*Y) -> Sum3/1
  Error/1 -> Subsystem1/1(X), Subsystem/2(Y)
  [Ki_IM] -> Subsystem1/2(Y)
  [Kp_IM] -> Subsystem/1(X)
  Sum3/1 -> PI/1
  En/1 -> Logical Operator/1, Subsystem1/3(En), Subsystem/3(En)
  Logical Operator/1 -> FF Int/2
  Constant2/1 -> FF Int/3
  Subsystem1/1(X*Y) -> FF Int/1
  FF Int/1 -> Sum3/2

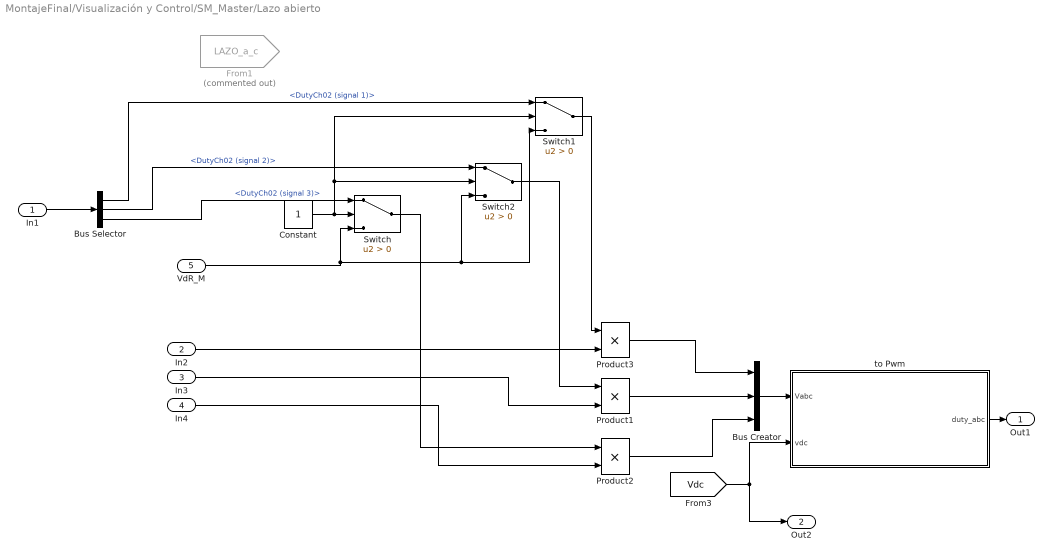
== system MontajeFinal/Visualización y Control/SM_Master/Lazo abierto  ==
  In1 : Inport
  In2 : Inport  Port=2
  In3 : Inport  Port=3
  In4 : Inport  Port=4
  VdR_M : Inport  Port=5
  Bus Creator : BusCreator  Inputs=3
  Bus Selector : BusSelector  OutputSignals=DutyCh02 (signal 1),DutyCh02 (signal 2),DutyCh02 (signal 3)
  Constant : Constant
  From1 : From  Commented=on  GotoTag=LAZO_a_c  TagVisibility=global
  Product1 : Product  RndMeth=Zero
  Product2 : Product  RndMeth=Zero
  Product3 : Product  RndMeth=Zero
  Switch : Switch  Criteria=u2 > Threshold  SaturateOnIntegerOverflow=off  InputSameDT=off
  Switch1 : Switch  Criteria=u2 > Threshold  SaturateOnIntegerOverflow=off  InputSameDT=off
  Switch2 : Switch  Criteria=u2 > Threshold  SaturateOnIntegerOverflow=off  InputSameDT=off
  to Pwm : Subsystem
      mask Display:
      | disp('Modulation');
      | port_label('input', 1, 'Vpwm');
      | port_label('input', 2, 'Vdc');
      | port_label('output', 1, 'duty');
  Out1 : Outport
  Out2 : Outport  Port=2
  wires:
  In3/1 -> Product1/2
  In4/1 -> Product2/2
  In2/1 -> Product3/2
  [Vdc] -> Out2/1, to Pwm/2(vdc)
  Product3/1 -> Bus Creator/1
  Product1/1 -> Bus Creator/2
  Product2/1 -> Bus Creator/3
  to Pwm/1(duty_abc) -> Out1/1
  Bus Creator/1 -> to Pwm/1(Vabc)
  In1/1 -> Bus Selector/1
  Bus Selector/3 -> Switch/1  "<DutyCh02 (signal 3)>"
  VdR_M/1 -> Switch1/3, Switch2/3, Switch/3
  Constant/1 -> Switch1/2, Switch2/2, Switch/2
  Switch/1 -> Product2/1
  Switch2/1 -> Product1/1
  Bus Selector/2 -> Switch2/1  "<DutyCh02 (signal 2)>"
  Bus Selector/1 -> Switch1/1  "<DutyCh02 (signal 1)>"
  Switch1/1 -> Product3/1

== system MontajeFinal/Visualización y Control/SM_Master/PWM ==
  A1 : Constant  Value=20
  B1 : Constant  Value=10080
  Bus Creator : BusCreator  Inputs=3
  Bus Creator2 : BusCreator  Inputs=3
  Bus Creator3 : BusCreator  Inputs=2
  "pwm " : Outport
  wires:
  Bus Creator2/1 -> Bus Creator3/1  "FreqPWMOut"
  Bus Creator/1 -> Bus Creator3/2  "DutyPWMOut"
  Bus Creator3/1 -> "pwm "/1  "PWMO_Ch00_07"
  A1/1 -> Bus Creator/2, Bus Creator/3, Bus Creator/1  "DutyCh02"
  B1/1 -> Bus Creator2/1, Bus Creator2/2, Bus Creator2/3  "FreqCh00"

== system MontajeFinal/Visualización y Control/SM_Master/Parametros de control ==
  Constant : Constant  Value=0.0655
  Constant1 : Constant  Value=22.739
  Constant2 : Constant  Value=20
  Constant3 : Constant  Value=50
  tag scope: Ki_IM=global, Ki_VM=global, Kp_IM=global, Kp_VM=global
  wires:
  Constant3/1 -> [Ki_IM]
  Constant1/1 -> [Ki_VM]
  Constant2/1 -> [Kp_IM]
  Constant/1 -> [Kp_VM]

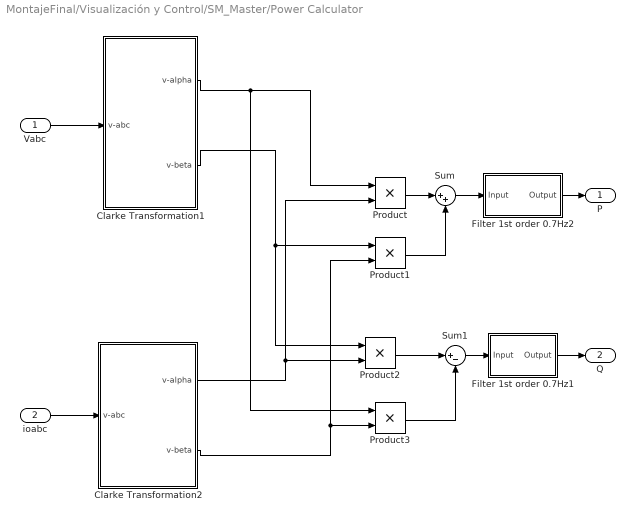
== system MontajeFinal/Visualización y Control/SM_Master/Power Calculator ==
  Vabc : Inport
  ioabc : Inport  Port=2
  Clarke Transformation1 : Subsystem
  Clarke Transformation2 : Subsystem
  Filter 1st order 0.7Hz1 : Subsystem  Tag=FilterWizardSubSystem
      settings: ErrorFcn=dspFilterRealizedInBasicElemsAlgLoopErrFcnCallback
  Filter 1st order 0.7Hz2 : Subsystem  Tag=FilterWizardSubSystem
      settings: ErrorFcn=dspFilterRealizedInBasicElemsAlgLoopErrFcnCallback
  Product{,1..3} (4 alike) : Product  RndMeth=Zero
  Sum : Sum  Inputs=|++
  Sum1 : Sum  Inputs=|+-
  P : Outport
  "Q " : Outport  Port=2
  wires:
  Vabc/1 -> Clarke Transformation1/1(v-abc)
  ioabc/1 -> Clarke Transformation2/1(v-abc)
  Product/1 -> Sum/1
  Product1/1 -> Sum/2
  Product2/1 -> Sum1/1
  Product3/1 -> Sum1/2
  Sum/1 -> Filter 1st order 0.7Hz2/1(Input)
  Sum1/1 -> Filter 1st order 0.7Hz1/1(Input)
  Clarke Transformation1/1(v-alpha) -> Product3/1, Product/1
  Clarke Transformation1/2(v-beta) -> Product1/1, Product2/1
  Clarke Transformation2/1(v-alpha) -> Product2/2, Product/2
  Clarke Transformation2/2(v-beta) -> Product3/2, Product1/2
  Filter 1st order 0.7Hz1/1(Output) -> "Q "/1
  Filter 1st order 0.7Hz2/1(Output) -> P/1

== system MontajeFinal/Visualización y Control/SM_Master/Subsystem2 ==
  In1 : Inport
  In2 : Inport  Port=2
  In3 : Inport  Port=3
  Constant3 : Constant  Value=0.8
  Demux5 : Demux  Outputs=3
  Gen Rampa : Subsystem
  Product3 : Product  RndMeth=Zero
  Three-phase Sine Wave : Sin  TimeSource=Use external signal  Phase=[0 -2*pi/3 2*pi/3]
  Out1 : Outport
  Out2 : Outport  Port=2
  Out3 : Outport  Port=3
  tag scope: wt=global
  wires:
  Demux5/1 -> Out1/1
  Product3/1 -> Demux5/1
  Demux5/2 -> Out2/1
  Three-phase Sine Wave/1 -> Product3/1
  Constant3/1 -> Product3/2  "<mod_index>"
  Demux5/3 -> Out3/1
  Gen Rampa/1("wt ") -> [wt], Three-phase Sine Wave/1
  In3/1 -> Gen Rampa/3(En)
  In2/1 -> Gen Rampa/2(Frec)
  In1/1 -> Gen Rampa/1(Fase)

== system MontajeFinal/Visualización y Control/SM_Master/Union señales  ==
  Mux1 : Mux  Inputs=3
  Mux5 : Mux  Inputs=3
  tag scope: Io_M=global, Vo_M=global
  wires:
  [Im_b] -> Mux5/2
  Mux5/1 -> [Io_M]
  [Im_c] -> Mux5/3
  [Vm_a] -> Mux1/1
  [Vm_c] -> Mux1/3
  [Im_a] -> Mux5/1
  Mux1/1 -> [Vo_M]
  [Vm_b] -> Mux1/2

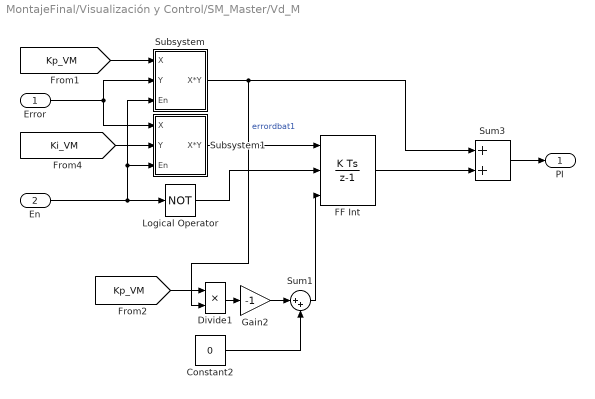
== system MontajeFinal/Visualización y Control/SM_Master/Vd_M ==
  Error : Inport
  En : Inport  Port=2
  Constant2 : Constant  Value=0
  Divide1 : Product  Inputs=**  OutDataTypeStr=Inherit: Same as first input
  FF Int : DiscreteIntegrator  ExternalReset=level  InitialConditionSource=external  InitialCondition=4  SampleTime=Ts  ICPrevOutput=DiscIntNeverNeededParam  ICPrevScaledInput=DiscIntNeverNeededParam
  Gain2 : Gain  Gain=-1
  Logical Operator : Logic  Operator=NOT  AllPortsSameDT=off  OutDataTypeStr=boolean
  Subsystem : Subsystem
  Subsystem1 : Subsystem
  Sum1 : Sum  Inputs=|++
  Sum3 : Sum  OutDataTypeStr=Inherit: Same as first input
  PI : Outport
  wires:
  Error/1 -> Subsystem1/1(X), Subsystem/2(Y)
  [Ki_VM] -> Subsystem1/2(Y)
  [Kp_VM] -> Subsystem/1(X)
  Sum3/1 -> PI/1
  En/1 -> Logical Operator/1, Subsystem1/3(En), Subsystem/3(En)
  Logical Operator/1 -> FF Int/2
  Gain2/1 -> Sum1/1
  [Kp_VM] -> Divide1/1
  Divide1/1 -> Gain2/1
  Subsystem/1(X*Y) -> Divide1/2, Sum3/1  "errordbat1"
  Sum1/1 -> FF Int/3
  Constant2/1 -> Sum1/2
  Subsystem1/1(X*Y) -> FF Int/1
  FF Int/1 -> Sum3/2

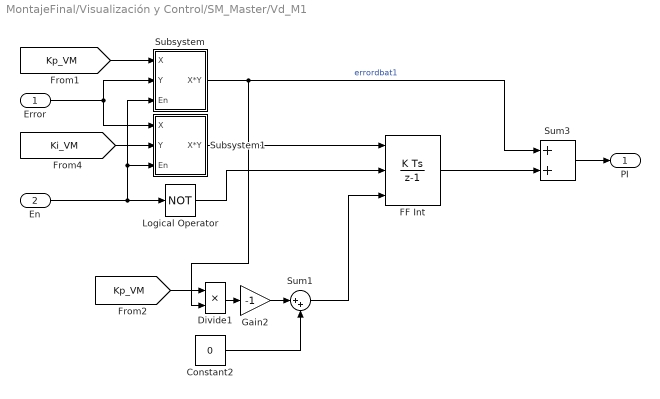
== system MontajeFinal/Visualización y Control/SM_Master/Vd_M1 ==
  Error : Inport
  En : Inport  Port=2
  Constant2 : Constant  Value=0
  Divide1 : Product  Inputs=**  OutDataTypeStr=Inherit: Same as first input
  FF Int : DiscreteIntegrator  ExternalReset=level  InitialConditionSource=external  InitialCondition=4  SampleTime=Ts  ICPrevOutput=DiscIntNeverNeededParam  ICPrevScaledInput=DiscIntNeverNeededParam
  Gain2 : Gain  Gain=-1
  Logical Operator : Logic  Operator=NOT  AllPortsSameDT=off  OutDataTypeStr=boolean
  Subsystem : Subsystem
  Subsystem1 : Subsystem
  Sum1 : Sum  Inputs=|++
  Sum3 : Sum  OutDataTypeStr=Inherit: Same as first input
  PI : Outport
  wires:
  Error/1 -> Subsystem1/1(X), Subsystem/2(Y)
  [Ki_VM] -> Subsystem1/2(Y)
  [Kp_VM] -> Subsystem/1(X)
  Sum3/1 -> PI/1
  En/1 -> Logical Operator/1, Subsystem1/3(En), Subsystem/3(En)
  Logical Operator/1 -> FF Int/2
  Gain2/1 -> Sum1/1
  [Kp_VM] -> Divide1/1
  Divide1/1 -> Gain2/1
  Subsystem/1(X*Y) -> Divide1/2, Sum3/1  "errordbat1"
  Sum1/1 -> FF Int/3
  Constant2/1 -> Sum1/2
  Subsystem1/1(X*Y) -> FF Int/1
  FF Int/1 -> Sum3/2

== system MontajeFinal/Visualización y Control/SM_Master/abc//dq_VM ==
  abc : Inport
  wt : Inport  Port=2
  Subsystem2 : Subsystem
  abc/alfabeta2 : Subsystem  mask{k=2/3}
  d : Outport
  Q : Outport  Port=2
  wires:
  abc/alfabeta2/1(alfa) -> Subsystem2/1(alfa)
  abc/alfabeta2/2(Beta) -> Subsystem2/2(beta)
  wt/1 -> Subsystem2/3(wt)
  Subsystem2/2(Q) -> Q/1
  abc/1 -> abc/alfabeta2/1(abc)
  Subsystem2/1(d) -> d/1

== system MontajeFinal/Visualización y Control/SM_Master/abc//dq_VM1 ==
  abc : Inport
  wt : Inport  Port=2
  Subsystem2 : Subsystem
  abc/alfabeta2 : Subsystem  mask{k=2/3}
  d : Outport
  Q : Outport  Port=2
  wires:
  Subsystem2/1(d) -> d/1
  abc/1 -> abc/alfabeta2/1(abc)
  Subsystem2/2(Q) -> Q/1
  wt/1 -> Subsystem2/3(wt)
  abc/alfabeta2/2(Beta) -> Subsystem2/2(beta)
  abc/alfabeta2/1(alfa) -> Subsystem2/1(alfa)

== system MontajeFinal/Visualización y Control/SM_Master/dq//abc ==
  d : Inport
  q : Inport  Port=2
  wt : Inport  Port=3
  Subsystem1 : Subsystem  mask{k=1}
  dq/alfabeta1 : Subsystem
  a : Outport
  b : Outport  Port=2
  c : Outport  Port=3
  wires:
  dq/alfabeta1/1(alfa) -> Subsystem1/1(alfa)
  dq/alfabeta1/2(beta) -> Subsystem1/2(beta)
  wt/1 -> dq/alfabeta1/3(wt)
  d/1 -> dq/alfabeta1/1(d)
  Subsystem1/1(a) -> a/1
  Subsystem1/3(c) -> c/1
  Subsystem1/2(b) -> b/1
  q/1 -> dq/alfabeta1/2(q)

== system MontajeFinal/Visualización y Control/SM_Master/to pwm_M ==
  In1 : Inport
  In2 : Inport  Port=2
  Bus Creator2 : BusCreator  Inputs=3
  Demux1 : Demux  Outputs=3
  Salida PWM : Subsystem
  Switch : Switch  Criteria=u2 > Threshold  SaturateOnIntegerOverflow=off  InputSameDT=off
  to Pwm1 : Subsystem
      mask Display:
      | disp('Modulation');
      | port_label('input', 1, 'Vpwm');
      | port_label('input', 2, 'Vdc');
      | port_label('output', 1, 'duty');
  wires:
  In1/1 -> to Pwm1/1(Vabc)
  Demux1/3 -> Bus Creator2/3
  Demux1/1 -> Bus Creator2/1
  In2/1 -> to Pwm1/2(vdc)
  Demux1/2 -> Bus Creator2/2
  Bus Creator2/1 -> Salida PWM/1("ciclo util ")
  [TEST] -> Switch/3
  [LAZO_a_c] -> Switch/2
  Switch/1 -> Demux1/1
  to Pwm1/1(duty_abc) -> Switch/1

== system MontajeFinal/Visualización y Control/SM_Master/Id_M/Subsystem ==
  X : Inport
  Y : Inport  Port=2
  En : Inport  Port=3
  Divide2 : Product  Inputs=**  OutDataTypeStr=Inherit: Same as first input
  Divide5 : Product  Inputs=**  OutDataTypeStr=Inherit: Same as first input
  X*Y : Outport
  wires:
  X/1 -> Divide2/1
  En/1 -> Divide5/2
  Divide2/1 -> Divide5/1
  Divide5/1 -> X*Y/1
  Y/1 -> Divide2/2

== system MontajeFinal/Visualización y Control/SM_Master/Id_M/Subsystem1 ==
  X : Inport
  Y : Inport  Port=2
  En : Inport  Port=3
  Divide2 : Product  Inputs=**  OutDataTypeStr=Inherit: Same as first input
  Divide5 : Product  Inputs=**  OutDataTypeStr=Inherit: Same as first input
  X*Y : Outport
  wires:
  X/1 -> Divide2/1
  En/1 -> Divide5/2
  Divide2/1 -> Divide5/1
  Divide5/1 -> X*Y/1
  Y/1 -> Divide2/2

== system MontajeFinal/Visualización y Control/SM_Master/Iq_M/Subsystem ==
  X : Inport
  Y : Inport  Port=2
  En : Inport  Port=3
  Divide2 : Product  Inputs=**  OutDataTypeStr=Inherit: Same as first input
  Divide5 : Product  Inputs=**  OutDataTypeStr=Inherit: Same as first input
  X*Y : Outport
  wires:
  X/1 -> Divide2/1
  En/1 -> Divide5/2
  Divide2/1 -> Divide5/1
  Divide5/1 -> X*Y/1
  Y/1 -> Divide2/2

== system MontajeFinal/Visualización y Control/SM_Master/Iq_M/Subsystem1 ==
  X : Inport
  Y : Inport  Port=2
  En : Inport  Port=3
  Divide2 : Product  Inputs=**  OutDataTypeStr=Inherit: Same as first input
  Divide5 : Product  Inputs=**  OutDataTypeStr=Inherit: Same as first input
  X*Y : Outport
  wires:
  X/1 -> Divide2/1
  En/1 -> Divide5/2
  Divide2/1 -> Divide5/1
  Divide5/1 -> X*Y/1
  Y/1 -> Divide2/2

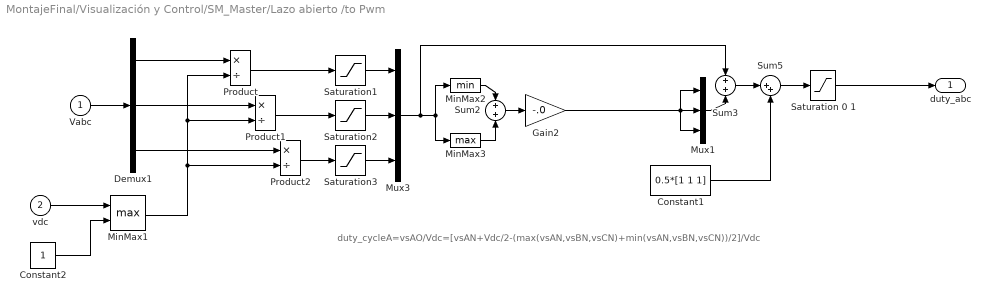
== system MontajeFinal/Visualización y Control/SM_Master/Lazo abierto /to Pwm ==
  note: duty_cycleA=vsAO/Vdc=[vsAN+Vdc/2-(max(vsAN,vsBN,vsCN)+min(vsAN,vsBN,vsCN))/2]/Vdc
  Vabc : Inport
  vdc : Inport  Port=2
  Constant1 : Constant  Value=0.5*[1 1 1]
  Constant2 : Constant
  Demux1 : Demux  Outputs=3
  Gain2 : Gain  Gain=-.0  SaturateOnIntegerOverflow=on  OutDataTypeStr=Inherit: Same as input  ParamDataTypeStr=Inherit: Same as input
  MinMax1 : MinMax  Function=max  Inputs=2  InputSameDT=on  SaturateOnIntegerOverflow=on
  MinMax2 : MinMax  InputSameDT=on  SaturateOnIntegerOverflow=on
  MinMax3 : MinMax  Function=max  InputSameDT=on  SaturateOnIntegerOverflow=on
  Mux1 : Mux  Inputs=3
  Mux3 : Mux  Inputs=3
  Product : Product  Inputs=*/  SaturateOnIntegerOverflow=on  OutDataTypeStr=Inherit: Same as first input
  Product1 : Product  Inputs=*/  SaturateOnIntegerOverflow=on  OutDataTypeStr=Inherit: Same as first input
  Product2 : Product  Inputs=*/  SaturateOnIntegerOverflow=on  OutDataTypeStr=Inherit: Same as first input
  Saturation 0 1 : Saturate  UpperLimit=0.98  LowerLimit=0.02
  Saturation1 : Saturate  UpperLimit=1/sqrt(3)  LowerLimit=-1/sqrt(3)
  Saturation2 : Saturate  UpperLimit=1/sqrt(3)  LowerLimit=-1/sqrt(3)
  Saturation3 : Saturate  UpperLimit=1/sqrt(3)  LowerLimit=-1/sqrt(3)
  Sum2 : Sum  InputSameDT=on  SaturateOnIntegerOverflow=on  OutDataTypeStr=Inherit: Same as first input
  Sum3 : Sum  InputSameDT=on  SaturateOnIntegerOverflow=on  OutDataTypeStr=Inherit: Same as first input
  Sum5 : Sum  Inputs=|++  InputSameDT=on  SaturateOnIntegerOverflow=on  OutDataTypeStr=Inherit: Same as first input
  duty_abc : Outport
  wires:
  Sum5/1 -> Saturation 0 1/1
  Mux3/1 -> MinMax3/1, MinMax2/1, Sum3/1
  MinMax3/1 -> Sum2/2
  MinMax2/1 -> Sum2/1
  Sum2/1 -> Gain2/1
  Gain2/1 -> Mux1/2, Mux1/3, Mux1/1
  Sum3/1 -> Sum5/1
  Constant1/1 -> Sum5/2
  Demux1/3 -> Product2/1
  Demux1/1 -> Product/1
  Saturation1/1 -> Mux3/1
  Saturation2/1 -> Mux3/2
  Saturation3/1 -> Mux3/3
  Product/1 -> Saturation1/1
  Product1/1 -> Saturation2/1
  Demux1/2 -> Product1/1
  Product2/1 -> Saturation3/1
  Saturation 0 1/1 -> duty_abc/1
  Mux1/1 -> Sum3/2
  vdc/1 -> MinMax1/1
  MinMax1/1 -> Product2/2, Product1/2, Product/2
  Constant2/1 -> MinMax1/2
  Vabc/1 -> Demux1/1

== system MontajeFinal/Visualización y Control/SM_Master/Power Calculator/Clarke Transformation1 ==
  v-abc : Inport
  Clarke to Beta : Fcn  Expr=0*u[1]+sqrt(1/2)*u[2]-sqrt(1/2)*u[3]
  Clarke to alpha : Fcn  Expr=sqrt(2/3)*u[1]-sqrt(1/6)*u[2]-sqrt(1/6)*u[3]
  v-alpha : Outport
  v-beta : Outport  Port=2
  wires:
  Clarke to Beta/1 -> v-beta/1
  Clarke to alpha/1 -> v-alpha/1
  v-abc/1 -> Clarke to Beta/1, Clarke to alpha/1

== system MontajeFinal/Visualización y Control/SM_Master/Power Calculator/Clarke Transformation2 ==
  v-abc : Inport
  Clarke to Beta : Fcn  Expr=0*u[1]+sqrt(1/2)*u[2]-sqrt(1/2)*u[3]
  Clarke to alpha : Fcn  Expr=sqrt(2/3)*u[1]-sqrt(1/6)*u[2]-sqrt(1/6)*u[3]
  v-alpha : Outport
  v-beta : Outport  Port=2
  wires:
  v-abc/1 -> Clarke to alpha/1, Clarke to Beta/1
  Clarke to alpha/1 -> v-alpha/1
  Clarke to Beta/1 -> v-beta/1

== system MontajeFinal/Visualización y Control/SM_Master/Power Calculator/Filter 1st order 0.7Hz1 ==
  Input : Inport
  Delay11 : Delay  DelayLength=1  InitialCondition=0
  SumA21 : Sum  Inputs=|+-  RndMeth=Nearest  SaturateOnIntegerOverflow=on  OutDataTypeStr=Inherit: Same as first input
  SumB21 : Sum  Inputs=|++  RndMeth=Nearest  SaturateOnIntegerOverflow=on  OutDataTypeStr=Inherit: Same as first input
  a(2)(1) : Gain  Gain=-0.99956027372226808  ParamDataTypeStr=float('double')  RndMeth=Nearest  SaturateOnIntegerOverflow=on  OutDataTypeStr=Inherit: Same as input
  s(1) : Gain  Gain=0.00021986313886602718  ParamDataTypeStr=float('double')  RndMeth=Nearest  SaturateOnIntegerOverflow=on  OutDataTypeStr=Inherit: Same as input
  Output : Outport
  wires:
  Delay11/1 -> SumB21/2, a(2)(1)/1
  a(2)(1)/1 -> SumA21/2
  SumB21/1 -> Output/1
  SumA21/1 -> Delay11/1, SumB21/1
  s(1)/1 -> SumA21/1
  Input/1 -> s(1)/1

== system MontajeFinal/Visualización y Control/SM_Master/Power Calculator/Filter 1st order 0.7Hz2 ==
  Input : Inport
  Delay11 : Delay  DelayLength=1  InitialCondition=0
  SumA21 : Sum  Inputs=|+-  RndMeth=Nearest  SaturateOnIntegerOverflow=on  OutDataTypeStr=Inherit: Same as first input
  SumB21 : Sum  Inputs=|++  RndMeth=Nearest  SaturateOnIntegerOverflow=on  OutDataTypeStr=Inherit: Same as first input
  a(2)(1) : Gain  Gain=-0.99956027372226808  ParamDataTypeStr=float('double')  RndMeth=Nearest  SaturateOnIntegerOverflow=on  OutDataTypeStr=Inherit: Same as input
  s(1) : Gain  Gain=0.00021986313886602718  ParamDataTypeStr=float('double')  RndMeth=Nearest  SaturateOnIntegerOverflow=on  OutDataTypeStr=Inherit: Same as input
  Output : Outport
  wires:
  Input/1 -> s(1)/1
  s(1)/1 -> SumA21/1
  SumA21/1 -> SumB21/1, Delay11/1
  SumB21/1 -> Output/1
  a(2)(1)/1 -> SumA21/2
  Delay11/1 -> a(2)(1)/1, SumB21/2

== system MontajeFinal/Visualización y Control/SM_Master/Subsystem2/Gen Rampa ==
  Fase : Inport
  Frec : Inport  Port=2
  En : Inport  Port=3
  Add1 : Sum
  Compare To Constant1 : simulink/Logic and Bit Operations/Compare To Constant  relop=>=  const=2*pi  OutDataTypeStr=boolean
  Gain : Gain  Gain=2*pi
  Gain6 : Gain  Gain=pi/180
  Integrator : Integrator  ExternalReset=rising
  Product : Product
  Unit Delay2 : UnitDelay  SampleTime=Ts  HasFrameUpgradeWarning=on
  "wt " : Outport
  wires:
  Unit Delay2/1 -> Integrator/2
  Add1/1 -> "wt "/1
  En/1 -> Product/2
  Gain6/1 -> Add1/1
  Compare To Constant1/1 -> Unit Delay2/1
  Fase/1 -> Gain6/1
  Gain/1 -> Product/1
  Product/1 -> Integrator/1
  Integrator/1 -> Add1/2, Compare To Constant1/1
  Frec/1 -> Gain/1
